simulink model "MG_DroopControl_ModeleSimplifie_pour_MPC"  (R2024b)
settings: Solver=ode4  StartTime=0.0  StopTime=900  FixedStep=1e-4  MaxStep=0.1  MinStep=0.001  RelTol=1e-3
undefined symbols (not defined in the file): f_nom, J, Kd, Pbat_max, Pg_nom, R, sigbuilder_block, Td, Te, Tn, w_nom
libraries: mpclib x1, spspowerguiLib x1
settings Model: Creator=atanno01  LastModifiedBy=euler
settings SolverCC: ZeroCrossAlgorithm=Adaptive
settings DataIOCC: SaveState=on
settings OptimizationCC: DefaultUnderspecifiedDataType=single  ReuseModelBlockBuffer=off
settings DebuggingCC: IgnoredZcDiagnostic=none
settings RTWCC: GPUComputeCapability=3.5

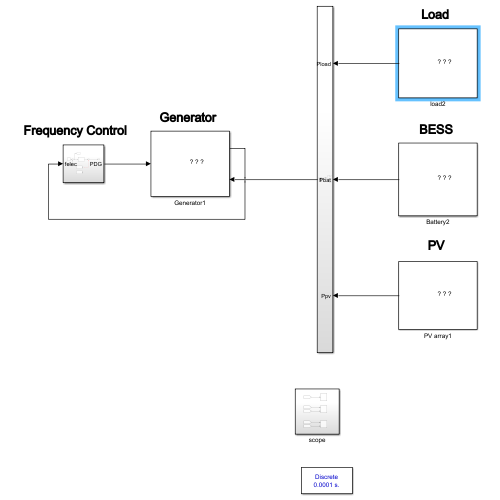
[thumbnail: Simulink's stored preview of the top-level diagram]
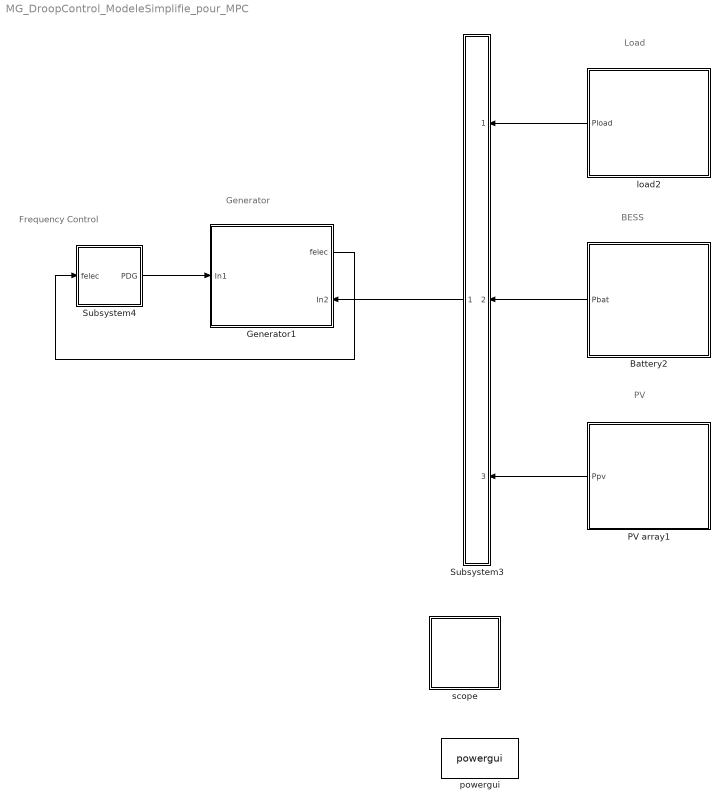
== system MG_DroopControl_ModeleSimplifie_pour_MPC ==
  note: PV
  note: Frequency Control
  note: BESS
  note: Generator
  note: Load
  Battery2 : Subsystem
      mask Display: image('C:\Users\atanno01\Desktop\General Documents\MATLAB Simulation\Microgrid MG\icons\Battt.png'); % Use "Edit Image" on toolstrip to change.
  Generator1 : Subsystem
      settings: PortSchema="{\"entries\":[{\"content\":{\"sides\":[{\"content\":{\"connectorIds\":[\"In1\"]},\"type\":\"ConnectorPlacement.EquallySpacedRectSide\",\"uuid\":\"72a34547-efe8-479e-a1ef-d23d1d343c7e\"},{\"content\":{\"connectorIds\":[\"Out1\",\"In2\"],\"side\":\"RIGHT\"},\"type\":\"ConnectorPlacement.EquallySpacedRectSide\",\"uuid\":\"b8cd4e31-6ecc-421d-a606-c424f5ade7de\"},{\"content\":{\"connectorIds\":[],\"side\":\"TOP\"},\"type\":\"ConnectorPlacement.EquallySpacedRectSide\",\"uuid\":\"cfef9a92-8723-48b3-9ba6-349d5d4d7378\"}]},\"type\":\"ConnectorPlacement.EquallySpacedConnector\",\"uuid\":\"d27d53b0-c096-42b6-9e9b-bfbc50f4b135\"}],\"packageUris\":[\"http://schema.mathworks.com/mf0/Connector/R2020b\"],\"version\":\"1.0\"}"
      mask Display: image('C:\Users\atanno01\Desktop\General Documents\MATLAB Simulation\Microgrid MG\icons\diesel1.png'); % Use "Edit Image" on toolstrip to change.
  PV array1 : Subsystem
      mask Display: image('C:\Users\atanno01\Desktop\General Documents\MATLAB Simulation\Microgrid MG\icons\PV3.png'); % Use "Edit Image" on toolstrip to change.
  Subsystem3 : Subsystem
  Subsystem4 : Subsystem
  load2 : Subsystem
      mask Display: image('C:\Users\atanno01\Desktop\General Documents\MATLAB Simulation\Microgrid MG\Microgrid test\icons\house.png'); % Use "Edit Image" on toolstrip to change.
  powergui : spspowerguiLib/powergui  Priority=1  SimulationMode=Discrete  SampleTime=0.0001  frequency=60  Iterations=50  frequencyindice=0  Pbase=1000e6  ErrMax=1e-4  UnitsV=kV  UnitsW=MW  buscounter=0  FunctionMessages=off  echomessages=off  EnableUseOfTLC=off  CurrentSourceSwitches=off  DisableSnubberDevices=off  DisableRonSwitches=off  DisableVfSwitches=off  DisplayEquations=off  AutomaticDiscreteSolvers=off  SolverType=Tustin/Backward Euler (TBE)  Interpol=off  ExternalGateDelay=off  methode=off  Ts=100  x0status=blocks  SPID=on  SwTol=0  HookPort=off  NonlinearTolerance=1e-4  nMaxIteration=100  ContinueOnMaxIteration=off  RestoreLinks=warning  ResistiveCurrentMeasurement=off  Frange=[0:2:500]  Ylog=off  Xlog=on  ShowGrid=off  save=off  variable=ZData  structure=0  ZoomFFT=off  StartTime=0.0  cycles=1  DisplayStyle=1  fundamental=60  FreqAxis=off  MaxFrequency=1000  frequencyindicesteady=1  RmsSteady=1  display=off
  scope : Subsystem
  wires:
  Subsystem4/1(PDG) -> Generator1/1(In1)
  Subsystem3/1(Out1) -> Generator1/2(In2)
  Generator1/1(felec) -> Subsystem4/1(felec)
  Battery2/1(Pbat) -> Subsystem3/2(Pbat)
  load2/1(Pload) -> Subsystem3/1(Pload)
  PV array1/1(Ppv) -> Subsystem3/3(Ppv)

== system MG_DroopControl_ModeleSimplifie_pour_MPC/Battery2 ==
  Battery Control : Subsystem
  Pbat : Outport
  tag scope: Pbat=global
  wires:
  Battery Control/1(Pbat ref) -> [Pbat], Pbat/1  "droop only"

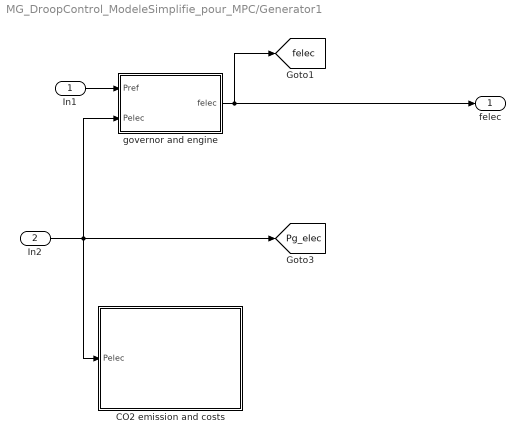
== system MG_DroopControl_ModeleSimplifie_pour_MPC/Generator1 ==
  In1 : Inport
  In2 : Inport  Port=2
  CO2 emission and costs : Subsystem
  governor and engine : Subsystem
  felec : Outport
  tag scope: Pg_elec=global, felec=global
  wires:
  In1/1 -> governor and engine/1(Pref)
  governor and engine/1(felec) -> felec/1, [felec]
  In2/1 -> CO2 emission and costs/1(Pelec), governor and engine/2(Pelec), [Pg_elec]

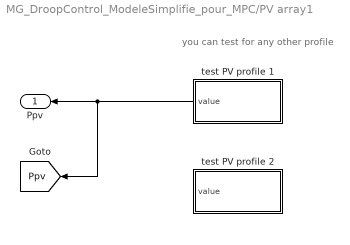
== system MG_DroopControl_ModeleSimplifie_pour_MPC/PV array1 ==
  note: you can test for any other profile
  test PV profile 1 : Subsystem  Tag=STV Subsys  LoadFcn=sigbuilder_block('load');  StartFcn=sigbuilder_block('start');  StopFcn=sigbuilder_block('stop');  ClipboardFcn=sigbuilder_block('clipboard');  mask(Sigbuilder block){tuvar=[0:10]}
      mask help: Simulink:masks:SigbuilderBlock_MD
      mask init:
      | if ~strcmp(get_param(bdroot(gcbh),'SimulationStatus'),'stopped') tuvar = sigbuilder_block('maskInit'); end
      settings: CopyFcn=sigbuilder_block('copy');  DeleteFcn=sigbuilder_block('delete');  ModelCloseFcn=sigbuilder_block('modelClose');  PreSaveFcn=sigbuilder_block('preSave');  PauseFcn=sigbuilder_block('pause');  ContinueFcn=sigbuilder_block('continue');  NameChangeFcn=sigbuilder_block('namechange');  OpenFcn=sigbuilder_block('open',[1271.25 -62.25 550.5 399.75 ]);  CloseFcn=sigbuilder_block('close');
      mask Display: plot(0, 0, 100, 100,[2, 2, 32, 32, 2], [68, 8, 8, 68, 68],[32, 2], [38, 38], [32, 19, 2],[53, 60, 44], [32, 17, 17, 2],[16, 16, 31, 31]);txt = getActiveGroup(gcbh);text(2, 100, txt,'verticalAlignment', 'top');
  test PV profile 2 : Subsystem  Tag=STV Subsys  LoadFcn=sigbuilder_block('load');  StartFcn=sigbuilder_block('start');  StopFcn=sigbuilder_block('stop');  ClipboardFcn=sigbuilder_block('clipboard');  mask(Sigbuilder block){tuvar=[0:10]}
      mask help: Simulink:masks:SigbuilderBlock_MD
      mask init:
      | if ~strcmp(get_param(bdroot(gcbh),'SimulationStatus'),'stopped') tuvar = sigbuilder_block('maskInit'); end
      settings: CopyFcn=sigbuilder_block('copy');  DeleteFcn=sigbuilder_block('delete');  ModelCloseFcn=sigbuilder_block('modelClose');  PreSaveFcn=sigbuilder_block('preSave');  PauseFcn=sigbuilder_block('pause');  ContinueFcn=sigbuilder_block('continue');  NameChangeFcn=sigbuilder_block('namechange');  OpenFcn=sigbuilder_block('open',[358.5 93 550.5 399.5 ]);  CloseFcn=sigbuilder_block('close');
      mask Display: plot(0, 0, 100, 100,[2, 2, 32, 32, 2], [68, 8, 8, 68, 68],[32, 2], [38, 38], [32, 19, 2],[53, 60, 44], [32, 17, 17, 2],[16, 16, 31, 31]);txt = getActiveGroup(gcbh);text(2, 100, txt,'verticalAlignment', 'top');
  Ppv : Outport
  tag scope: Ppv=global
  wires:
  test PV profile 1/1(value) -> [Ppv], Ppv/1

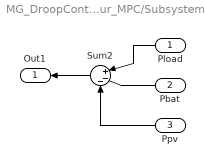
== system MG_DroopControl_ModeleSimplifie_pour_MPC/Subsystem3 ==
  Pload : Inport
  Pbat : Inport  Port=2
  Ppv : Inport  Port=3
  Sum2 : Sum  Inputs=|+--
  Out1 : Outport
  wires:
  Sum2/1 -> Out1/1
  Pload/1 -> Sum2/1
  Pbat/1 -> Sum2/2
  Ppv/1 -> Sum2/3

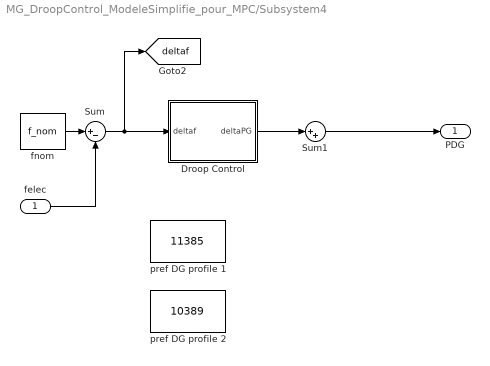
== system MG_DroopControl_ModeleSimplifie_pour_MPC/Subsystem4 ==
  felec : Inport
  Droop Control : Subsystem
  Sum : Sum  Inputs=|+-
  Sum1 : Sum  Inputs=|++
  fnom : Constant  Value=f_nom
  pref DG profile 1 : Constant  Value=11385
  pref DG profile 2 : Constant  Value=10389
  PDG : Outport
  tag scope: deltaf=global
  wires:
  Droop Control/1(deltaPG) -> Sum1/1
  Sum/1 -> [deltaf], Droop Control/1(deltaf)
  felec/1 -> Sum/2
  Sum1/1 -> PDG/1
  fnom/1 -> Sum/1
  ? -> Sum1/2

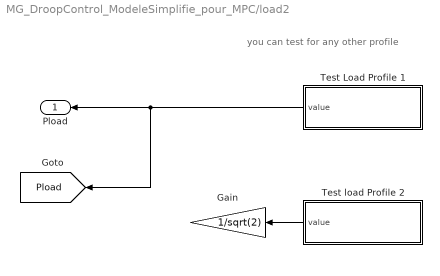
== system MG_DroopControl_ModeleSimplifie_pour_MPC/load2 ==
  note: you can test for any other profile
  Gain : Gain  Gain=1/sqrt(2)
  Test Load Profile 1 : Subsystem  Tag=STV Subsys  LoadFcn=sigbuilder_block('load');  StartFcn=sigbuilder_block('start');  StopFcn=sigbuilder_block('stop');  ClipboardFcn=sigbuilder_block('clipboard');  mask(Sigbuilder block){tuvar=[0:10]}
      mask help: Simulink:masks:SigbuilderBlock_MD
      mask init:
      | if ~strcmp(get_param(bdroot(gcbh),'SimulationStatus'),'stopped') tuvar = sigbuilder_block('maskInit'); end
      settings: CopyFcn=sigbuilder_block('copy');  DeleteFcn=sigbuilder_block('delete');  ModelCloseFcn=sigbuilder_block('modelClose');  PreSaveFcn=sigbuilder_block('preSave');  PauseFcn=sigbuilder_block('pause');  ContinueFcn=sigbuilder_block('continue');  NameChangeFcn=sigbuilder_block('namechange');  OpenFcn=sigbuilder_block('open',[437.6 153 550.4 359.25 ]);  CloseFcn=sigbuilder_block('close');
      mask Display: plot(0, 0, 100, 100,[2, 2, 32, 32, 2], [68, 8, 8, 68, 68],[32, 2], [38, 38], [32, 19, 2],[53, 60, 44], [32, 17, 17, 2],[16, 16, 31, 31]);txt = getActiveGroup(gcbh);text(2, 100, txt,'verticalAlignment', 'top');
  Test load Profile 2 : Subsystem  Tag=STV Subsys  LoadFcn=sigbuilder_block('load');  StartFcn=sigbuilder_block('start');  StopFcn=sigbuilder_block('stop');  ClipboardFcn=sigbuilder_block('clipboard');  mask(Sigbuilder block){tuvar=[0:10]}
      mask help: Simulink:masks:SigbuilderBlock_MD
      mask init:
      | if ~strcmp(get_param(bdroot(gcbh),'SimulationStatus'),'stopped') tuvar = sigbuilder_block('maskInit'); end
      settings: CopyFcn=sigbuilder_block('copy');  DeleteFcn=sigbuilder_block('delete');  ModelCloseFcn=sigbuilder_block('modelClose');  PreSaveFcn=sigbuilder_block('preSave');  PauseFcn=sigbuilder_block('pause');  ContinueFcn=sigbuilder_block('continue');  NameChangeFcn=sigbuilder_block('namechange');  OpenFcn=sigbuilder_block('open',[384 96.75 550.5 399.75 ]);  CloseFcn=sigbuilder_block('close');
      mask Display: plot(0, 0, 100, 100,[2, 2, 32, 32, 2], [68, 8, 8, 68, 68],[32, 2], [38, 38], [32, 19, 2],[53, 60, 44], [32, 17, 17, 2],[16, 16, 31, 31]);txt = getActiveGroup(gcbh);text(2, 100, txt,'verticalAlignment', 'top');
  Pload : Outport
  tag scope: Pload=global
  wires:
  Test Load Profile 1/1(value) -> [Pload], Pload/1
  Test load Profile 2/1(value) -> Gain/1

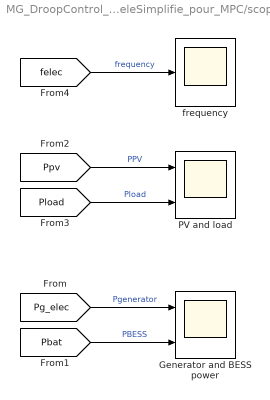
== system MG_DroopControl_ModeleSimplifie_pour_MPC/scope ==
  Generator and BESS power : Scope  NumInputPorts=2
  PV and load : Scope  NumInputPorts=2
  frequency : Scope
  wires:
  [Pg_elec] -> Generator and BESS power/1  "Pgenerator"
  [Pbat] -> Generator and BESS power/2  "PBESS"
  [Ppv] -> PV and load/1  "PPV"
  [Pload] -> PV and load/2  "Pload"
  [felec] -> frequency/1  "frequency"

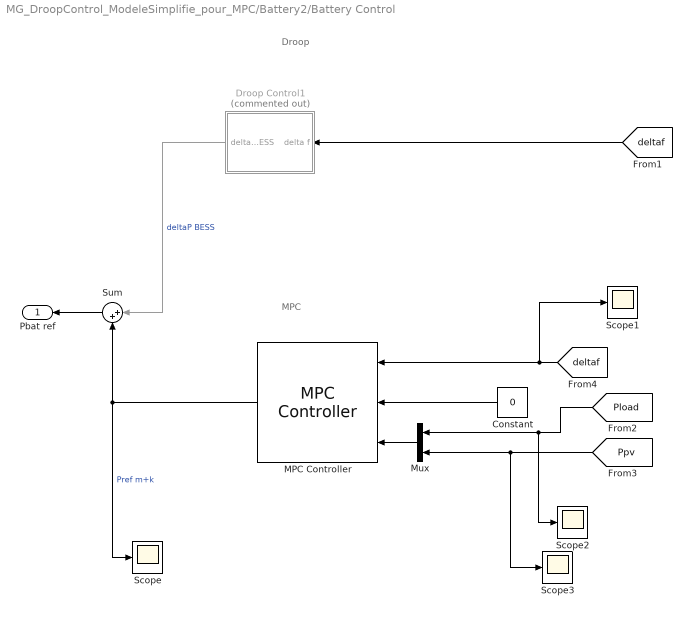
== system MG_DroopControl_ModeleSimplifie_pour_MPC/Battery2/Battery Control ==
  note: Droop
  note: MPC
  Constant : Constant  Value=0
  Droop Control1 : Subsystem  Commented=on
  MPC Controller : mpclib/MPC Controller  SCDEnableBlockLinearizationSpecification=on  mpcobj=mpcobj  is_multiple=0  enable_value=0  return_u0=off  updateMPCinCallerWorkspace=on  md_inport=on  mv_inport=off  uref_inport=off  return_cost=off  return_mvseq=off  return_qpstatus=off  return_xseq=off  return_state=off  return_ovseq=off  state_inport=off  umin_inport=off  umax_inport=off  ymin_inport=off  ymax_inport=off  cc_inport=off  ywt_inport=off  uwt_inport=off  duwt_inport=off  rhoeps_inport=off  pm_inport=off  MaximumP=10  HorizonChoice=FixedHorizon  n_ts=1  n_p=360  n_mv=1  n_md=2  n_ud=0  n_mo=1  n_uo=0  BlockDataType=double  SampleTimeInherited=off  switch_inport=off
  Mux : Mux  Inputs=2
  Scope{,1..3} (4 alike) : Scope
  Sum : Sum  Inputs=|++
  Pbat ref : Outport
  wires:
  [deltaf] -> Droop Control1/1(delta f)
  Droop Control1/1(deltaP BESS) -> Sum/1  "deltaP BESS"
  Sum/1 -> Pbat ref/1
  MPC Controller/1 -> Scope/1, Sum/2  "Pref m+k"
  [Pload] -> Scope2/1, Mux/1
  [Ppv] -> Scope3/1, Mux/2
  Mux/1 -> MPC Controller/3
  Constant/1 -> MPC Controller/2
  [deltaf] -> Scope1/1, MPC Controller/1

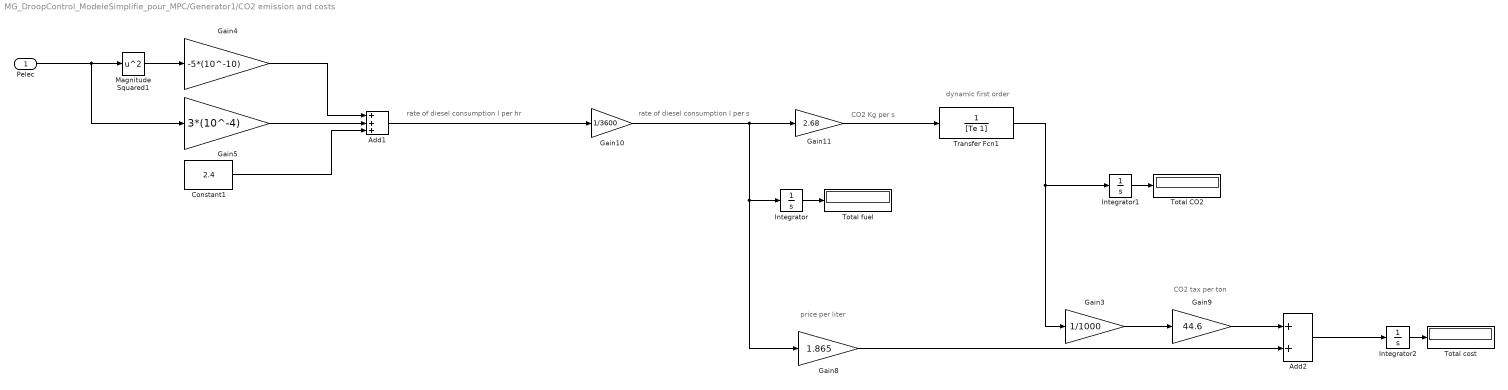
== system MG_DroopControl_ModeleSimplifie_pour_MPC/Generator1/CO2 emission and costs ==
  note: rate of diesel consumption l per hr
  note: CO2 tax per ton
  note: rate of diesel consumption l per s
  note: dynamic first order
  note: price per liter
  note: CO2 Kg per s
  Pelec : Inport
  Add1 : Sum  Inputs=+++
  Add2 : Sum
  Constant1 : Constant  Value=2.4
  Gain10 : Gain  Gain=1/3600
  Gain11 : Gain  Gain=2.68
  Gain3 : Gain  Gain=1/1000
  Gain4 : Gain  Gain=-5*(10^-10)
  Gain5 : Gain  Gain=3*(10^-4)
  Gain8 : Gain  Gain=1.865
  Gain9 : Gain  Gain=44.6
  Integrator : Integrator
  Integrator1 : Integrator
  Integrator2 : Integrator
  Magnitude Squared1 : Math  Operator=square
  Total CO2 : Display
  Total cost : Display
  Total fuel : Display
  Transfer Fcn1 : TransferFcn  Denominator=[Te 1]
  wires:
  Pelec/1 -> Magnitude Squared1/1, Gain5/1
  Gain4/1 -> Add1/1
  Constant1/1 -> Add1/3
  Magnitude Squared1/1 -> Gain4/1
  Gain5/1 -> Add1/2
  Integrator1/1 -> Total CO2/1
  Integrator2/1 -> Total cost/1
  Gain8/1 -> Add2/2
  Transfer Fcn1/1 -> Integrator1/1, Gain3/1
  Integrator/1 -> Total fuel/1
  Add2/1 -> Integrator2/1
  Gain3/1 -> Gain9/1
  Gain10/1 -> Gain8/1, Integrator/1, Gain11/1
  Gain9/1 -> Add2/1
  Gain11/1 -> Transfer Fcn1/1
  Add1/1 -> Gain10/1

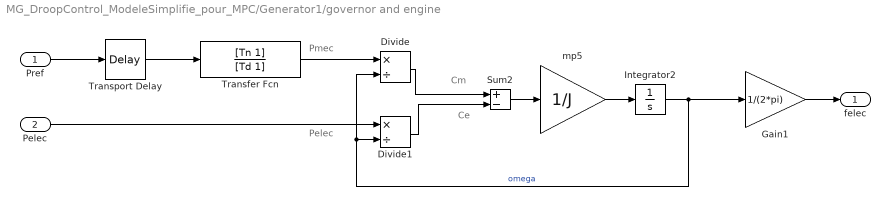
== system MG_DroopControl_ModeleSimplifie_pour_MPC/Generator1/governor and engine ==
  note: Ce
  note: Cm
  note: Pmec
  note: Pelec
  Pref : Inport
  Pelec : Inport  Port=2
  Divide : Product  Inputs=*/
  Divide1 : Product  Inputs=*/
  Gain1 : Gain  Gain=1/(2*pi)
  Integrator2 : Integrator  InitialCondition=w_nom
  Sum2 : Sum  Inputs=+-
  Transfer Fcn : TransferFcn  Numerator=[Tn 1]  Denominator=[Td 1]
  Transport Delay : TransportDelay  DelayTime=Te
  mp5 : Gain  Gain=1/J
  felec : Outport
  wires:
  Pelec/1 -> Divide1/1
  Divide1/1 -> Sum2/2
  Sum2/1 -> mp5/1
  mp5/1 -> Integrator2/1
  Divide/1 -> Sum2/1
  Transfer Fcn/1 -> Divide/1
  Pref/1 -> Transport Delay/1
  Transport Delay/1 -> Transfer Fcn/1
  Gain1/1 -> felec/1
  Integrator2/1 -> Divide1/2, Divide/2, Gain1/1  "omega"

== system MG_DroopControl_ModeleSimplifie_pour_MPC/PV array1/test PV profile 1 ==
  Demux : Demux  Tag=STV Demux  Outputs=1
      settings: DisplayOption=none
  FromWs : FromWorkspace  Tag=STV FromWs  VariableName=tuvar
      SigBuilderData=|
      | common.afterFinalStr = 'Extrapolate'
      | common.sampleTime = 0
      | dataSet.timeRange = [0 900]
      | dataSet.name = 'PV_Power_Real'
      | sbobj.Groups.Name = 'PV_Power_Real'
      | sbobj.Groups.Signals.Name = 'value'
      | sbobj.Groups.Signals.XData = [0 60 120 180 240 300 360 420 480 540 600 660 720 780 840 900]
      | sbobj.Groups.Signals.YData = [4420 4379 4355 4292 4096 4095 4171 4196 4181 4170 4103 3996 3947 3895 3930 3802]
      | sbobj.Groups.TimeRange = [0 900]
  value : Outport  Tag=STV Outport
  wires:
  Demux/1 -> value/1
  FromWs/1 -> Demux/1

== system MG_DroopControl_ModeleSimplifie_pour_MPC/PV array1/test PV profile 2 ==
  Demux : Demux  Tag=STV Demux  Outputs=1
      settings: DisplayOption=none
  FromWs : FromWorkspace  Tag=STV FromWs  VariableName=tuvar
      SigBuilderData=|
      | common.afterFinalStr = 'Extrapolate'
      | common.sampleTime = 0
      | dataSet.timeRange = [0 900]
      | dataSet.name = 'PV real'
      | sbobj.Groups.Name = 'PV real'
      | sbobj.Groups.Signals.Name = 'value'
      | sbobj.Groups.Signals.XData = [0 60 120 180 240 300 360 420 480 540 600 660 720 780 840 900]
      | sbobj.Groups.Signals.YData = [898 1066 1114 1377 1462 1534 1607 1653 2001 2268 2481 2645 2808 2929 3076 3240]
      | sbobj.Groups.TimeRange = [0 900]
  value : Outport  Tag=STV Outport
  wires:
  Demux/1 -> value/1
  FromWs/1 -> Demux/1

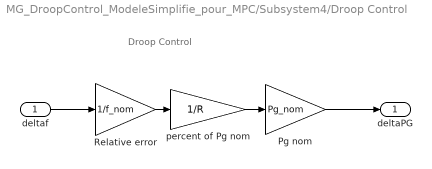
== system MG_DroopControl_ModeleSimplifie_pour_MPC/Subsystem4/Droop Control ==
  note: Droop Control
  deltaf : Inport
  Pg nom : Gain  Gain=Pg_nom
  Relative error : Gain  Gain=1/f_nom
  percent of Pg nom : Gain  Gain=1/R
  deltaPG : Outport
  wires:
  deltaf/1 -> Relative error/1
  percent of Pg nom/1 -> Pg nom/1
  Relative error/1 -> percent of Pg nom/1
  Pg nom/1 -> deltaPG/1

== system MG_DroopControl_ModeleSimplifie_pour_MPC/load2/Test Load Profile 1 ==
  Demux : Demux  Tag=STV Demux  Outputs=1
      settings: DisplayOption=none
  FromWs : FromWorkspace  Tag=STV FromWs  VariableName=tuvar
      SigBuilderData=|
      | common.afterFinalStr = 'Extrapolate'
      | common.sampleTime = 0
      | dataSet.timeRange = [0 900]
      | dataSet.name = 'Load_Power_Real'
      | sbobj.Groups.Name = 'Load_Power_Real'
      | sbobj.Groups.Signals.Name = 'value'
      | sbobj.Groups.Signals.XData = [0 60 120 180 240 300 360 420 480 540 600 660 720 780 840 900]
      | sbobj.Groups.Signals.YData = [30975 31230 31825 31825 31825 31825 32420 32505 32420 32505 32420 32335 32335 32335 32335 32335]
      | sbobj.Groups.TimeRange = [0 900]
  value : Outport  Tag=STV Outport
  wires:
  Demux/1 -> value/1
  FromWs/1 -> Demux/1

== system MG_DroopControl_ModeleSimplifie_pour_MPC/load2/Test load Profile 2 ==
  Demux : Demux  Tag=STV Demux  Outputs=1
      settings: DisplayOption=none
  FromWs : FromWorkspace  Tag=STV FromWs  VariableName=tuvar
      SigBuilderData=|
      | common.afterFinalStr = 'Extrapolate'
      | common.sampleTime = 0
      | dataSet.timeRange = [0 900]
      | dataSet.name = 'Load real'
      | sbobj.Groups.Name = 'Load real'
      | sbobj.Groups.Signals.Name = 'value'
      | sbobj.Groups.Signals.XData = [0 60 120 180 240 300 360 420 480 540 600 660 720 780 840 900]
      | sbobj.Groups.Signals.YData = [11631 11546 12141 12566 12566 12481 12481 12481 12481 12481 12481 12481 12481 12481 12396 12396]
      | sbobj.Groups.TimeRange = [0 900]
  value : Outport  Tag=STV Outport
  wires:
  Demux/1 -> value/1
  FromWs/1 -> Demux/1

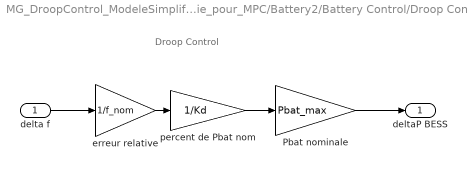
== system MG_DroopControl_ModeleSimplifie_pour_MPC/Battery2/Battery Control/Droop Control1 ==
  note: Droop Control
  delta f : Inport
  Pbat nominale : Gain  Gain=Pbat_max
  erreur relative : Gain  Gain=1/f_nom
  percent de Pbat nom : Gain  Gain=1/Kd
  deltaP BESS : Outport
  wires:
  delta f/1 -> erreur relative/1
  percent de Pbat nom/1 -> Pbat nominale/1
  erreur relative/1 -> percent de Pbat nom/1
  Pbat nominale/1 -> deltaP BESS/1
